simulink model "ISController"  (R2018a)
settings: Solver=FixedStepDiscrete  StartTime=0.0  StopTime=12  FixedStep=0.001  RelTol=1e-3  EnableMultiTasking=on
values from neighbouring files (symbols this model uses):
  Bx_ash_f = 11.7    [ISData.m]    (also in pacjeka_params.m)
  Bx_ash_r = 11.1    [ISData.m]    (also in pacjeka_params.m)
  Bx_snow_f = 10.2    [ISData.m]    (also in pacjeka_params.m)
  Bx_snow_r = 9.71    [ISData.m]    (also in pacjeka_params.m)
  By_ash_f = 8.86    [ISData.m]    (also in pacjeka_params.m)
  By_ash_r = 9.30    (= 9.3)    [ISData.m]    (also in pacjeka_params.m)
  By_snow_f = 19.1    [ISData.m]    (also in pacjeka_params.m)
  By_snow_r = 20.0    (= 20)    [ISData.m]    (also in pacjeka_params.m)
  Cx_ash_f = 1.69    [ISData.m]    (also in pacjeka_params.m)
  Cx_ash_r = 1.69    [ISData.m]    (also in pacjeka_params.m)
  Cx_snow_f = 1.96    [ISData.m]    (also in pacjeka_params.m)
  Cx_snow_r = 1.96    [ISData.m]    (also in pacjeka_params.m)
  Cy_ash_f = 1.19    [ISData.m]    (also in pacjeka_params.m)
  Cy_ash_r = 1.19    [ISData.m]    (also in pacjeka_params.m)
  Cy_snow_f = 0.550    (= 0.55)    [ISData.m]    (also in pacjeka_params.m)
  Cy_snow_r = 0.550    (= 0.55)    [ISData.m]    (also in pacjeka_params.m)
  D_phi = 16000    [ISData.m]    (also in IS_2impulse.m; IS_3impulse.m; IS_4impulse.m; InputShaper.m)
  D_theta = 30960    [ISData.m]    (also in IS_2impulse.m; IS_3impulse.m; IS_4impulse.m; InputShaper.m)
  delta_r = 0    [ISData.m]    (also in IS_2impulse.m; IS_3impulse.m; IS_4impulse.m; InputShaper.m)
  DLCTest = [0 0 0 0 0 0 0 0 0 0 0 0 ... (12003 elements, 12003x1)]    [DLCTest.mat]
  epsilon = 0.4    [ISData.m]    (also in IS_2impulse.m; IS_3impulse.m; IS_4impulse.m; InputShaper.m)
  Ex_ash_f = 0.377    [ISData.m]    (also in pacjeka_params.m)
  Ex_ash_r = 0.362    [ISData.m]    (also in pacjeka_params.m)
  Ex_snow_f = 0.651    [ISData.m]    (also in pacjeka_params.m)
  Ex_snow_r = 0.624    [ISData.m]    (also in pacjeka_params.m)
  Ey_ash_f = -1.21    [ISData.m]    (also in pacjeka_params.m)
  Ey_ash_r = -1.11    [ISData.m]    (also in pacjeka_params.m)
  Ey_snow_f = -2.1    [ISData.m]    (also in pacjeka_params.m)
  Ey_snow_r = -1.93    [ISData.m]    (also in pacjeka_params.m)
  g = 9.81    [ISData.m]    (also in IS_2impulse.m; IS_3impulse.m; IS_4impulse.m; InputShaper.m)
  h = 0.5    [ISData.m]    (also in IS_2impulse.m; IS_3impulse.m; IS_4impulse.m; InputShaper.m)
  Iw = 4    [ISData.m]    (also in IS_2impulse.m; IS_3impulse.m; IS_4impulse.m; InputShaper.m)
  Ixx = 602.1923    [ISData.m]    (also in IS_2impulse.m; IS_3impulse.m; IS_4impulse.m; InputShaper.m)
  Iyy = 2.7370e+03    (= 2737)    [ISData.m]    (also in IS_2impulse.m; IS_3impulse.m; IS_4impulse.m; InputShaper.m)
  Izz = 3070    [ISData.m]    (also in IS_2impulse.m; IS_3impulse.m; IS_4impulse.m; InputShaper.m)
  K_phi = 178000    [ISData.m]    (also in IS_2impulse.m; IS_3impulse.m; IS_4impulse.m; InputShaper.m)
  K_theta = 363540    [ISData.m]    (also in IS_2impulse.m; IS_3impulse.m; IS_4impulse.m; InputShaper.m)
  l_f = 1.2110    (= 1.211)    [ISData.m]    (also in IS_2impulse.m; IS_3impulse.m; IS_4impulse.m; InputShaper.m)
  l_r = 1.4590    (= 1.459)    [ISData.m]    (also in IS_2impulse.m; IS_3impulse.m; IS_4impulse.m; InputShaper.m)
  m = 1830    [ISData.m]    (also in IS_2impulse.m; IS_3impulse.m; IS_4impulse.m; InputShaper.m)
  mu_x_ash_f = 1.20    (= 1.2)    [ISData.m]    (also in pacjeka_params.m)
  mu_x_ash_r = 1.20    (= 1.2)    [ISData.m]    (also in pacjeka_params.m)
  mu_x_snow_f = 0.407    [ISData.m]    (also in pacjeka_params.m)
  mu_x_snow_r = 0.409    [ISData.m]    (also in pacjeka_params.m)
  mu_y_ash_f = 0.935    [ISData.m]    (also in pacjeka_params.m)
  mu_y_ash_r = 0.961    [ISData.m]    (also in pacjeka_params.m)
  mu_y_snow_f = 0.383    [ISData.m]    (also in pacjeka_params.m)
  mu_y_snow_r = 0.394    [ISData.m]    (also in pacjeka_params.m)
  omega0 = Vx0/Rw    (= 64.7813411079)    [ISData.m]    (also in IS_2impulse.m = 74.1; IS_3impulse.m = 74.1; IS_4impulse.m = 74.1; InputShaper.m = 74.0666666667)
  road = 1    [ISData.m]    (also in IS_2impulse.m; IS_3impulse.m; IS_4impulse.m; InputShaper.m)
  Rw = 0.3430    (= 0.343)    [ISData.m]    (also in IS_2impulse.m = 0.3; IS_3impulse.m = 0.3; IS_4impulse.m = 0.3; InputShaper.m = 0.3)
  thetaSW_actual = [thetaSW_actual, deltaSW]    [IS_2impulse.m]    (also in InputShaper.m; InputShaper2.m; thetaSW_IS_L.mat = [0 0 0 0 0 0 0 0 0 0 0 0 ... (12003 elements, 1x12003)]; thetaSW_IS_NL.mat = [0 0 0 0 0 0 0 0 0 0 0 0 ... (12003 elements, 1x12003)])
  Ts = 0.001    [ISData.m]    (also in IS_2impulse.m; IS_3impulse.m; IS_4impulse.m; InputShaper.m)
  Tsmall = 0.001    [ISData.m]    (also in IS_2impulse.m; IS_3impulse.m; IS_4impulse.m; InputShaper.m)
  Vx0 = 22.22    [ISData.m]    (also in IS_2impulse.m = states(3); IS_3impulse.m = states(3); IS_4impulse.m = states(3); InputShaper.m = states(3))
  w = 0.7700    (= 0.77)    [ISData.m]    (also in IS_2impulse.m; IS_3impulse.m; IS_4impulse.m; InputShaper.m)
libraries: simulink x2
(part 1 of 4)
settings Model: ExtModeTrigDuration=10000  Creator=srivats  LastModifiedBy=srivats
settings SolverCC: PositivePriorityOrder=on
settings RTWCC: SystemTargetFile=quarc_win64.tlc  TemplateMakefile=quarc_default_tmf  Description=QUARC Win64 Target
settings STFCustomTargetCC: TargetPreCompLibLocation=C:\PROGRA~3\QUARC\lib\2018a\win64\release  TargetLangStandard=C99 (ISO)  ConcurrentExecutionCompliant=on  SystemTargetFile=quarc_win64.tlc
settings GRTTargetCC: TargetPreCompLibLocation=C:\PROGRA~3\QUARC\lib\2018a\win64\release  ParMdlRefBuildCompliant=off  CompOptLevelCompliant=off  CombineOutputUpdateFcns=off  MatFileLogging=off  CPPClassGenCompliant=off  GRTInterface=on  UseToolchainInfoCompliant=off  ExtMode=on  ExtModeMexFile=quarc_comm

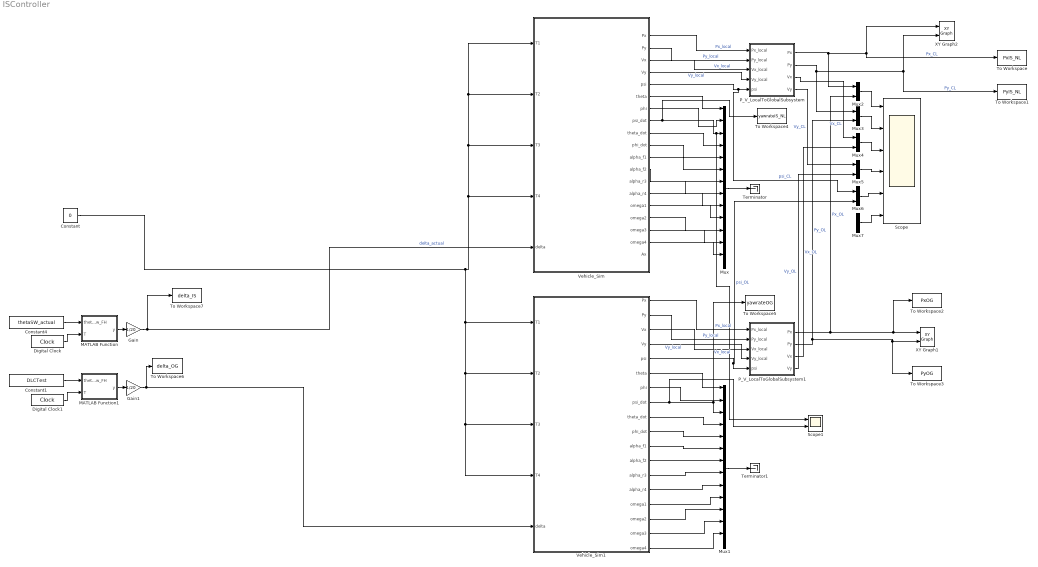
== system ISController ==
  Constant : Constant  Value=0
  Constant1 : Constant  Value=DLCTest
  Constant4 : Constant  Value=thetaSW_actual
  Digital Clock : DigitalClock  SampleTime=0.001
  Digital Clock1 : DigitalClock  SampleTime=0.001
  Gain : Gain  Gain=1/20
  Gain1 : Gain  Gain=1/20
  MATLAB Function : MATLAB Function  TreatAsAtomicUnit=on
  MATLAB Function1 : MATLAB Function  TreatAsAtomicUnit=on
  Mux : Mux  Inputs=14
  Mux1 : Mux  Inputs=14
  Mux{2..7} (6 alike) : Mux  Inputs=2
  P_V_LocalToGlobalSubsystem : Subsystem
  P_V_LocalToGlobalSubsystem1 : Subsystem
  Scope : Scope  NumInputPorts=6
  Scope1 : Scope  NumInputPorts=2
  Terminator : Terminator
  Terminator1 : Terminator
  To Workspace : ToWorkspace  VariableName=PxIS_NL  SaveFormat=Timeseries  SampleTime=-1
  To Workspace1 : ToWorkspace  VariableName=PyIS_NL  SaveFormat=Timeseries  SampleTime=-1
  To Workspace2 : ToWorkspace  VariableName=PxOG  SaveFormat=Timeseries  SampleTime=-1
  To Workspace3 : ToWorkspace  VariableName=PyOG  SaveFormat=Timeseries  SampleTime=-1
  To Workspace4 : ToWorkspace  VariableName=yawrateIS_NL  SaveFormat=Timeseries  SampleTime=-1
  To Workspace5 : ToWorkspace  VariableName=yawrateOG  SaveFormat=Timeseries  SampleTime=-1
  To Workspace6 : ToWorkspace  VariableName=delta_OG  SaveFormat=Timeseries  SampleTime=-1
  To Workspace7 : ToWorkspace  VariableName=delta_IS  SaveFormat=Timeseries  SampleTime=-1
  Vehicle_Sim : Subsystem
  Vehicle_Sim1 : Subsystem
  XY Graph1 : simulink/Sinks/XY Graph  xmin=0  xmax=700  ymin=-10  ymax=10  st=-1
  XY Graph2 : simulink/Sinks/XY Graph  xmin=0  xmax=700  ymin=-10  ymax=10  st=-1
  wires:
  Constant4/1 -> MATLAB Function/1(theta_sw_FH)
  Digital Clock/1 -> MATLAB Function/2(T)
  Vehicle_Sim1/10(phi_dot) -> Mux1/5
  Vehicle_Sim1/18(omega4) -> Mux1/13
  Vehicle_Sim1/7(phi) -> Mux1/2
  Vehicle_Sim/10(phi_dot) -> Mux/5
  Mux4/1 -> Scope/3
  Mux5/1 -> Scope/4
  P_V_LocalToGlobalSubsystem/4(Vy) -> Mux5/1  "Vy_CL"
  P_V_LocalToGlobalSubsystem1/3(Vx) -> Mux4/2  "Vx_OL"
  Mux2/1 -> Scope/1
  Vehicle_Sim1/15(omega1) -> Mux1/10
  Mux7/1 -> Scope/6
  Vehicle_Sim/17(omega3) -> Mux/12
  Mux6/1 -> Scope/5
  Vehicle_Sim1/14(alpha_r4) -> Mux1/9
  P_V_LocalToGlobalSubsystem1/2(Py) -> XY Graph1/2, To Workspace3/1, Mux3/2  "Py_OL"
  P_V_LocalToGlobalSubsystem1/4(Vy) -> Mux5/2  "Vy_OL"
  Vehicle_Sim/8(psi_dot) -> To Workspace4/1, Scope1/1, Mux/3
  Mux3/1 -> Scope/2
  P_V_LocalToGlobalSubsystem1/1(Px) -> Mux2/2, To Workspace2/1, XY Graph1/1  "Px_OL"
  Vehicle_Sim1/5(psi) -> Mux6/2, P_V_LocalToGlobalSubsystem1/5(psi)  "psi_OL"
  Vehicle_Sim1/12(alpha_f2) -> Mux1/7
  Vehicle_Sim/9(theta_dot) -> Mux/4
  Vehicle_Sim1/16(omega2) -> Mux1/11
  Vehicle_Sim/13(alpha_r3) -> Mux/8
  P_V_LocalToGlobalSubsystem/1(Px) -> XY Graph2/1, To Workspace/1, Mux2/1  "Px_CL"
  Constant/1 -> Vehicle_Sim1/4(T4), Vehicle_Sim1/3(T3), Vehicle_Sim1/2(T2), Vehicle_Sim1/1(T1), Vehicle_Sim/2(T2), Vehicle_Sim/1(T1), Vehicle_Sim/3(T3), Vehicle_Sim/4(T4)
  Vehicle_Sim/18(omega4) -> Mux/13
  Vehicle_Sim1/8(psi_dot) -> Scope1/2, To Workspace5/1, Mux1/3
  Mux1/1 -> Terminator1/1
  Vehicle_Sim/12(alpha_f2) -> Mux/7
  Vehicle_Sim1/17(omega3) -> Mux1/12
  Vehicle_Sim/16(omega2) -> Mux/11
  Vehicle_Sim1/6(theta) -> Mux1/1
  Vehicle_Sim1/13(alpha_r3) -> Mux1/8
  Vehicle_Sim1/4(Vy) -> P_V_LocalToGlobalSubsystem1/4(Vy_local)  "Vy_local"
  Vehicle_Sim1/2(Py) -> P_V_LocalToGlobalSubsystem1/2(Py_local)  "Py_local"
  Vehicle_Sim/3(Vx) -> P_V_LocalToGlobalSubsystem/3(Vx_local)  "Vx_local"
  Vehicle_Sim/5(psi) -> Mux6/1, P_V_LocalToGlobalSubsystem/5(psi)  "psi_CL"
  Vehicle_Sim/1(Px) -> P_V_LocalToGlobalSubsystem/1(Px_local)  "Px_local"
  Mux/1 -> Terminator/1
  P_V_LocalToGlobalSubsystem/2(Py) -> XY Graph2/2, To Workspace1/1, Mux3/1  "Py_CL"
  Vehicle_Sim/7(phi) -> Mux/2
  Vehicle_Sim1/3(Vx) -> P_V_LocalToGlobalSubsystem1/3(Vx_local)  "Vx_local"
  Vehicle_Sim/14(alpha_r4) -> Mux/9
  Vehicle_Sim1/11(alpha_f1) -> Mux1/6
  Vehicle_Sim/2(Py) -> P_V_LocalToGlobalSubsystem/2(Py_local)  "Py_local"
  P_V_LocalToGlobalSubsystem/3(Vx) -> Mux4/1  "Vx_CL"
  Vehicle_Sim/15(omega1) -> Mux/10
  Vehicle_Sim1/1(Px) -> P_V_LocalToGlobalSubsystem1/1(Px_local)  "Px_local"
  Vehicle_Sim1/9(theta_dot) -> Mux1/4
  Vehicle_Sim/4(Vy) -> P_V_LocalToGlobalSubsystem/4(Vy_local)  "Vy_local"
  Vehicle_Sim/6(theta) -> Mux/1
  Vehicle_Sim/11(alpha_f1) -> Mux/6
  MATLAB Function/1(y) -> Gain/1
  Gain/1 -> To Workspace7/1, Vehicle_Sim/5("delta ")  "delta_actual"
  MATLAB Function1/1(y) -> Gain1/1
  Constant1/1 -> MATLAB Function1/1(theta_sw_FH)
  Digital Clock1/1 -> MATLAB Function1/2(T)
  Gain1/1 -> To Workspace6/1, Vehicle_Sim1/5("delta ")

== system ISController/P_V_LocalToGlobalSubsystem ==
  Px_local : Inport  OutDataTypeStr=double  SampleTime=Ts
  Py_local : Inport  Port=2  OutDataTypeStr=double  SampleTime=Ts
  Vx_local : Inport  Port=3  OutDataTypeStr=double  SampleTime=Ts
  Vy_local : Inport  Port=4  OutDataTypeStr=double  SampleTime=Ts
  psi : Inport  Port=5  OutDataTypeStr=double  SampleTime=Ts
  Add : Sum  Inputs=+-
  Add1 : Sum
  Add2 : Sum  Inputs=+-
  Add3 : Sum
  Cos : Trigonometry  Operator=cos
  Product{,1..7} (8 alike) : Product
  Sin : Trigonometry
  Px : Outport  OutDataTypeStr=double  SampleTime=Ts
  Py : Outport  Port=2  OutDataTypeStr=double  SampleTime=Ts
  Vx : Outport  Port=3  OutDataTypeStr=double  SampleTime=Ts
  Vy : Outport  Port=4  OutDataTypeStr=double  SampleTime=Ts
  wires:
  Px_local/1 -> Product6/1, Product4/1  "Px_local"
  Py_local/1 -> Product7/1, Product5/1  "Py_local"
  Vx_local/1 -> Product2/1, Product/2  "Vx_local"
  Product5/1 -> Add2/2
  Product4/1 -> Add2/1
  Add2/1 -> Px/1  "Px"
  Product7/1 -> Add3/2
  Vy_local/1 -> Product3/1, Product1/2  "Vy_local"
  psi/1 -> Sin/1, Cos/1  "psi"
  Cos/1 -> Product3/2, Product/1, Product7/2, Product4/2  "cosPsi"
  Add3/1 -> Py/1  "Py"
  Product2/1 -> Add1/1
  Product1/1 -> Add/2
  Add/1 -> Vx/1  "Vx"
  Add1/1 -> Vy/1  "Vy"
  Product6/1 -> Add3/1
  Product3/1 -> Add1/2
  Product/1 -> Add/1
  Sin/1 -> Product2/2, Product1/1, Product6/2, Product5/2  "sinPsi"

== system ISController/P_V_LocalToGlobalSubsystem1 ==
  Px_local : Inport  OutDataTypeStr=double  SampleTime=Ts
  Py_local : Inport  Port=2  OutDataTypeStr=double  SampleTime=Ts
  Vx_local : Inport  Port=3  OutDataTypeStr=double  SampleTime=Ts
  Vy_local : Inport  Port=4  OutDataTypeStr=double  SampleTime=Ts
  psi : Inport  Port=5  OutDataTypeStr=double  SampleTime=Ts
  Add : Sum  Inputs=+-
  Add1 : Sum
  Add2 : Sum  Inputs=+-
  Add3 : Sum
  Cos : Trigonometry  Operator=cos
  Product{,1..7} (8 alike) : Product
  Sin : Trigonometry
  Px : Outport  OutDataTypeStr=double  SampleTime=Ts
  Py : Outport  Port=2  OutDataTypeStr=double  SampleTime=Ts
  Vx : Outport  Port=3  OutDataTypeStr=double  SampleTime=Ts
  Vy : Outport  Port=4  OutDataTypeStr=double  SampleTime=Ts
  wires:
  Px_local/1 -> Product6/1, Product4/1  "Px_local"
  Py_local/1 -> Product7/1, Product5/1  "Py_local"
  Vx_local/1 -> Product2/1, Product/2  "Vx_local"
  Product5/1 -> Add2/2
  Product4/1 -> Add2/1
  Add2/1 -> Px/1  "Px"
  Product7/1 -> Add3/2
  Vy_local/1 -> Product3/1, Product1/2  "Vy_local"
  psi/1 -> Sin/1, Cos/1  "psi"
  Cos/1 -> Product3/2, Product/1, Product7/2, Product4/2  "cosPsi"
  Add3/1 -> Py/1  "Py"
  Product2/1 -> Add1/1
  Product1/1 -> Add/2
  Add/1 -> Vx/1  "Vx"
  Add1/1 -> Vy/1  "Vy"
  Product6/1 -> Add3/1
  Product3/1 -> Add1/2
  Product/1 -> Add/1
  Sin/1 -> Product2/2, Product1/1, Product6/2, Product5/2  "sinPsi"

== system ISController/Vehicle_Sim ==
  T1 : Inport  OutDataTypeStr=double  SampleTime=Ts
  T2 : Inport  Port=2  OutDataTypeStr=double  SampleTime=Ts
  T3 : Inport  Port=3  OutDataTypeStr=double  SampleTime=Ts
  T4 : Inport  Port=4  OutDataTypeStr=double  SampleTime=Ts
  "delta " : Inport  Port=5
  Add1 : Sum
  Add2 : Sum
  Delay2 : Delay  DelayLength=1  SampleTime=Tsmall
  Delay3 : Delay  DelayLength=1  SampleTime=Tsmall
  Demux : Demux  Outputs=11
  Demux1 : Demux
  Gain1 : Gain  Gain=Tsmall
  Gain2 : Gain  Gain=Tsmall
  Mux : Mux  Inputs=11
      settings: DisplayOption=signals
  Mux1 : Mux
      settings: DisplayOption=signals
  Vehicle_model : Subsystem
  Vx_delay : Delay  DelayLength=1  InitialCondition=Vx0  SampleTime=Tsmall
  omega_delay : Delay  DelayLength=1  InitialCondition=omega0*ones(4,1)  SampleTime=Tsmall
  otherstates_delay : Delay  DelayLength=1  InitialCondition=zeros(11,1)  SampleTime=Tsmall
  Px : Outport  OutDataTypeStr=double  SampleTime=Tsmall
  Py : Outport  Port=2  OutDataTypeStr=double  SampleTime=Tsmall
  Vx : Outport  Port=3  OutDataTypeStr=double  SampleTime=Tsmall
  Vy : Outport  Port=4  OutDataTypeStr=double  SampleTime=Tsmall
  psi : Outport  Port=5  OutDataTypeStr=double  SampleTime=Tsmall
  theta : Outport  Port=6  OutDataTypeStr=double  SampleTime=Tsmall
  phi : Outport  Port=7  OutDataTypeStr=double  SampleTime=Tsmall
  psi_dot : Outport  Port=8  OutDataTypeStr=double  SampleTime=Tsmall
  theta_dot : Outport  Port=9  OutDataTypeStr=double  SampleTime=Tsmall
  phi_dot : Outport  Port=10  OutDataTypeStr=double  SampleTime=Tsmall
  alpha_f1 : Outport  Port=11  OutDataTypeStr=double  SampleTime=Tsmall
  alpha_f2 : Outport  Port=12  OutDataTypeStr=double  SampleTime=Tsmall
  alpha_r3 : Outport  Port=13  OutDataTypeStr=double  SampleTime=Tsmall
  alpha_r4 : Outport  Port=14  OutDataTypeStr=double  SampleTime=Tsmall
  omega1 : Outport  Port=15  OutDataTypeStr=double  SampleTime=Tsmall
  omega2 : Outport  Port=16  OutDataTypeStr=double  SampleTime=Tsmall
  omega3 : Outport  Port=17  OutDataTypeStr=double  SampleTime=Tsmall
  omega4 : Outport  Port=18  OutDataTypeStr=double  SampleTime=Tsmall
  Ax : Outport  Port=19
  wires:
  Vehicle_model/14(theta_next) -> Mux/9  "theta_next"
  Vehicle_model/12(psi_next) -> Mux/7  "psi_next"
  Vehicle_model/11(psi_dot_next) -> Mux/6  "psi_dot_next"
  Vehicle_model/15(phi_dot_next) -> Mux/10  "phi_dot_next"
  Mux/1 -> otherstates_delay/1
  Vehicle_model/3(alpha_f1_next) -> Mux/2  "alpha_f1_next"
  Vehicle_model/5(alpha_r3_next) -> Mux/4  "alpha_r3_next"
  Vehicle_model/9(omega3_next) -> Mux1/3  "omega3_next"
  Vehicle_model/8(omega2_next) -> Mux1/2  "omega2_next"
  Vehicle_model/13(theta_dot_next) -> Mux/8  "theta_dot_next"
  Vehicle_model/4(alpha_f2_next) -> Mux/3  "alpha_f2_next"
  Vehicle_model/6(alpha_r4_next) -> Mux/5  "alpha_r4_next"
  Vehicle_model/10(omega4_next) -> Mux1/4  "omega4_next"
  Vehicle_model/1(Vx_next) -> Vx_delay/1  "Vx_next"
  Demux/1 -> Gain2/1, Vy/1, Vehicle_model/6(Vy_curr)
  Vehicle_model/7(omega1_next) -> Mux1/1  "omega1_next"
  Demux1/3 -> omega3/1, Vehicle_model/13(omega3_curr)
  Demux/5 -> Vehicle_model/10(alpha_r4_curr), alpha_r4/1
  Demux/8 -> theta_dot/1, Vehicle_model/17(theta_dot_curr)
  Vehicle_model/16(phi_next) -> Mux/11  "phi_next"
  Vehicle_model/2(Vy_next) -> Mux/1  "Vy_next"
  T1/1 -> Vehicle_model/1(T1)
  Add2/1 -> Delay3/1
  Delay3/1 -> Py/1, Add2/2  "Py_curr"
  Add1/1 -> Delay2/1  "Px_next"
  Delay2/1 -> Px/1, Add1/2  "Px_curr"
  Gain1/1 -> Add1/1
  Gain2/1 -> Add2/1
  T3/1 -> Vehicle_model/3(T3)
  T4/1 -> Vehicle_model/4(T4)
  T2/1 -> Vehicle_model/2(T2)
  otherstates_delay/1 -> Demux/1
  Demux/4 -> Vehicle_model/9(alpha_r3_curr), alpha_r3/1
  Demux/11 -> phi/1, Vehicle_model/19(phi_curr)
  Demux/2 -> Vehicle_model/7(alpha_f1_curr), alpha_f1/1
  Demux/3 -> Vehicle_model/8(alpha_f2_curr), alpha_f2/1
  Demux1/4 -> omega4/1, Vehicle_model/14(omega4_curr)
  Demux/7 -> psi/1, Vehicle_model/16(psi_curr)
  Demux/9 -> theta/1, Vehicle_model/18(theta_curr)
  Demux/10 -> phi_dot/1, Vehicle_model/20(phi_dot_curr)
  Demux/6 -> psi_dot/1, Vehicle_model/15(psi_dot_curr)
  Demux1/2 -> omega2/1, Vehicle_model/12(omega2_curr)
  Vx_delay/1 -> Vx/1, Vehicle_model/5(Vx_curr), Gain1/1
  Demux1/1 -> omega1/1, Vehicle_model/11(omega1_curr)
  Mux1/1 -> omega_delay/1
  omega_delay/1 -> Demux1/1
  "delta "/1 -> Vehicle_model/21(delta)
  Vehicle_model/17(Ax) -> Ax/1

== system ISController/Vehicle_Sim1 ==
  T1 : Inport  OutDataTypeStr=double  SampleTime=Ts
  T2 : Inport  Port=2  OutDataTypeStr=double  SampleTime=Ts
  T3 : Inport  Port=3  OutDataTypeStr=double  SampleTime=Ts
  T4 : Inport  Port=4  OutDataTypeStr=double  SampleTime=Ts
  "delta " : Inport  Port=5
  Add1 : Sum
  Add2 : Sum
  Delay2 : Delay  DelayLength=1  SampleTime=Tsmall
  Delay3 : Delay  DelayLength=1  SampleTime=Tsmall
  Demux : Demux  Outputs=11
  Demux1 : Demux
  Gain1 : Gain  Gain=Tsmall
  Gain2 : Gain  Gain=Tsmall
  Mux : Mux  Inputs=11
      settings: DisplayOption=signals
  Mux1 : Mux
      settings: DisplayOption=signals
  Vehicle_model : Subsystem
  Vx_delay : Delay  DelayLength=1  InitialCondition=Vx0  SampleTime=Tsmall
  omega_delay : Delay  DelayLength=1  InitialCondition=omega0*ones(4,1)  SampleTime=Tsmall
  otherstates_delay : Delay  DelayLength=1  InitialCondition=zeros(11,1)  SampleTime=Tsmall
  Px : Outport  OutDataTypeStr=double  SampleTime=Tsmall
  Py : Outport  Port=2  OutDataTypeStr=double  SampleTime=Tsmall
  Vx : Outport  Port=3  OutDataTypeStr=double  SampleTime=Tsmall
  Vy : Outport  Port=4  OutDataTypeStr=double  SampleTime=Tsmall
  psi : Outport  Port=5  OutDataTypeStr=double  SampleTime=Tsmall
  theta : Outport  Port=6  OutDataTypeStr=double  SampleTime=Tsmall
  phi : Outport  Port=7  OutDataTypeStr=double  SampleTime=Tsmall
  psi_dot : Outport  Port=8  OutDataTypeStr=double  SampleTime=Tsmall
  theta_dot : Outport  Port=9  OutDataTypeStr=double  SampleTime=Tsmall
  phi_dot : Outport  Port=10  OutDataTypeStr=double  SampleTime=Tsmall
  alpha_f1 : Outport  Port=11  OutDataTypeStr=double  SampleTime=Tsmall
  alpha_f2 : Outport  Port=12  OutDataTypeStr=double  SampleTime=Tsmall
  alpha_r3 : Outport  Port=13  OutDataTypeStr=double  SampleTime=Tsmall
  alpha_r4 : Outport  Port=14  OutDataTypeStr=double  SampleTime=Tsmall
  omega1 : Outport  Port=15  OutDataTypeStr=double  SampleTime=Tsmall
  omega2 : Outport  Port=16  OutDataTypeStr=double  SampleTime=Tsmall
  omega3 : Outport  Port=17  OutDataTypeStr=double  SampleTime=Tsmall
  omega4 : Outport  Port=18  OutDataTypeStr=double  SampleTime=Tsmall
  wires:
  Vehicle_model/14(theta_next) -> Mux/9  "theta_next"
  Vehicle_model/12(psi_next) -> Mux/7  "psi_next"
  Vehicle_model/11(psi_dot_next) -> Mux/6  "psi_dot_next"
  Vehicle_model/15(phi_dot_next) -> Mux/10  "phi_dot_next"
  Mux/1 -> otherstates_delay/1
  Vehicle_model/3(alpha_f1_next) -> Mux/2  "alpha_f1_next"
  Vehicle_model/5(alpha_r3_next) -> Mux/4  "alpha_r3_next"
  Vehicle_model/9(omega3_next) -> Mux1/3  "omega3_next"
  Vehicle_model/8(omega2_next) -> Mux1/2  "omega2_next"
  Vehicle_model/13(theta_dot_next) -> Mux/8  "theta_dot_next"
  Vehicle_model/4(alpha_f2_next) -> Mux/3  "alpha_f2_next"
  Vehicle_model/6(alpha_r4_next) -> Mux/5  "alpha_r4_next"
  Vehicle_model/10(omega4_next) -> Mux1/4  "omega4_next"
  Vehicle_model/1(Vx_next) -> Vx_delay/1  "Vx_next"
  Demux/1 -> Gain2/1, Vy/1, Vehicle_model/6(Vy_curr)
  Vehicle_model/7(omega1_next) -> Mux1/1  "omega1_next"
  Demux1/3 -> omega3/1, Vehicle_model/13(omega3_curr)
  Demux/5 -> Vehicle_model/10(alpha_r4_curr), alpha_r4/1
  Demux/8 -> theta_dot/1, Vehicle_model/17(theta_dot_curr)
  Vehicle_model/16(phi_next) -> Mux/11  "phi_next"
  Vehicle_model/2(Vy_next) -> Mux/1  "Vy_next"
  T1/1 -> Vehicle_model/1(T1)
  Add2/1 -> Delay3/1
  Delay3/1 -> Py/1, Add2/2  "Py_curr"
  Add1/1 -> Delay2/1  "Px_next"
  Delay2/1 -> Px/1, Add1/2  "Px_curr"
  Gain1/1 -> Add1/1
  Gain2/1 -> Add2/1
  T3/1 -> Vehicle_model/3(T3)
  T4/1 -> Vehicle_model/4(T4)
  T2/1 -> Vehicle_model/2(T2)
  otherstates_delay/1 -> Demux/1
  Demux/4 -> Vehicle_model/9(alpha_r3_curr), alpha_r3/1
  Demux/11 -> phi/1, Vehicle_model/19(phi_curr)
  Demux/2 -> Vehicle_model/7(alpha_f1_curr), alpha_f1/1
  Demux/3 -> Vehicle_model/8(alpha_f2_curr), alpha_f2/1
  Demux1/4 -> omega4/1, Vehicle_model/14(omega4_curr)
  Demux/7 -> psi/1, Vehicle_model/16(psi_curr)
  Demux/9 -> theta/1, Vehicle_model/18(theta_curr)
  Demux/10 -> phi_dot/1, Vehicle_model/20(phi_dot_curr)
  Demux/6 -> psi_dot/1, Vehicle_model/15(psi_dot_curr)
  Demux1/2 -> omega2/1, Vehicle_model/12(omega2_curr)
  Vx_delay/1 -> Vx/1, Vehicle_model/5(Vx_curr), Gain1/1
  Demux1/1 -> omega1/1, Vehicle_model/11(omega1_curr)
  Mux1/1 -> omega_delay/1
  omega_delay/1 -> Demux1/1
  "delta "/1 -> Vehicle_model/21(delta)

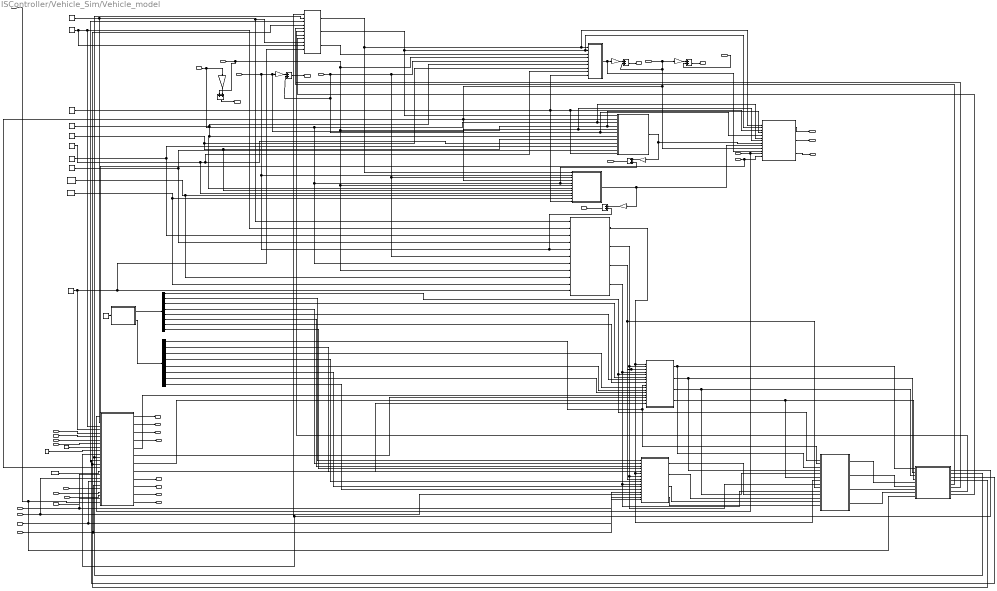
== system ISController/Vehicle_Sim/Vehicle_model ==
  T1 : Inport  OutDataTypeStr=double  SampleTime=Ts
  T2 : Inport  Port=2  OutDataTypeStr=double  SampleTime=Ts
  T3 : Inport  Port=3  OutDataTypeStr=double  SampleTime=Ts
  T4 : Inport  Port=4  OutDataTypeStr=double  SampleTime=Ts
  Vx_curr : Inport  Port=5  OutDataTypeStr=double  SampleTime=Tsmall
  Vy_curr : Inport  Port=6  OutDataTypeStr=double  SampleTime=Tsmall
  alpha_f1_curr : Inport  Port=7  OutDataTypeStr=double  SampleTime=Tsmall
  alpha_f2_curr : Inport  Port=8  OutDataTypeStr=double  SampleTime=Tsmall
  alpha_r3_curr : Inport  Port=9  OutDataTypeStr=double  SampleTime=Tsmall
  alpha_r4_curr : Inport  Port=10  OutDataTypeStr=double  SampleTime=Tsmall
  omega1_curr : Inport  Port=11  OutDataTypeStr=double  SampleTime=Tsmall
  omega2_curr : Inport  Port=12  OutDataTypeStr=double  SampleTime=Tsmall
  omega3_curr : Inport  Port=13  OutDataTypeStr=double  SampleTime=Tsmall
  omega4_curr : Inport  Port=14  OutDataTypeStr=double  SampleTime=Tsmall
  psi_dot_curr : Inport  Port=15  OutDataTypeStr=double  SampleTime=Tsmall
  psi_curr : Inport  Port=16  OutDataTypeStr=double  SampleTime=Tsmall
  theta_dot_curr : Inport  Port=17  OutDataTypeStr=double  SampleTime=Tsmall
  theta_curr : Inport  Port=18  OutDataTypeStr=double  SampleTime=Tsmall
  phi_curr : Inport  Port=19  OutDataTypeStr=double  SampleTime=Tsmall
  phi_dot_curr : Inport  Port=20  OutDataTypeStr=double  SampleTime=Tsmall
  delta : Inport  Port=21  OutDataTypeStr=double  SampleTime=Tsmall
  Add{,1..5} (6 alike) : Sum
  D_phi : Constant  Value=D_phi
  D_theta : Constant  Value=D_theta
  Demux1 : Demux  Outputs=8
  Demux2 : Demux  Outputs=8
  F_M_subsystem : Subsystem
  Fx0_Subsystem : Subsystem
  Fy0_Subsystem : Subsystem
  Fy0_to_Fy_subsystem : Subsystem
  Fz_Subsystem : Subsystem
  Gain{,1..5} (6 alike) : Gain  Gain=Tsmall
  Iw : Constant  Value=Iw
  Ixx : Constant  Value=Ixx
  Iyy : Constant  Value=Iyy
  Izz : Constant  Value=Izz
  K_phi : Constant  Value=K_phi
  K_theta : Constant  Value=K_theta
  Pacjeka_parameters_Subsystem : Subsystem
  Rw : Constant  Value=Rw
  Vx_Vy_Subsystem : Subsystem
  epsilon : Constant  Value=epsilon
  h : Constant  Value=h
  l_f : Constant  Value=l_f
  l_r : Constant  Value=l_r
  local_to_global_Fx_Fy_Subsystem : Subsystem
  omega_alpha_and_k_values_subsystem : Subsystem
  phi_subsystem : Subsystem
  psi_subsystem : Subsystem
  surface : Constant  Value=road
  theta_subsystem : Subsystem
  w : Constant  Value=w
  Vx_next : Outport  OutDataTypeStr=double  SampleTime=Tsmall
  Vy_next : Outport  Port=2  OutDataTypeStr=double  SampleTime=Tsmall
  alpha_f1_next : Outport  Port=3  OutDataTypeStr=double  SampleTime=Tsmall
  alpha_f2_next : Outport  Port=4  OutDataTypeStr=double  SampleTime=Tsmall
  alpha_r3_next : Outport  Port=5  OutDataTypeStr=double  SampleTime=Tsmall
  alpha_r4_next : Outport  Port=6  OutDataTypeStr=double  SampleTime=Tsmall
  omega1_next : Outport  Port=7  OutDataTypeStr=double  SampleTime=Tsmall
  omega2_next : Outport  Port=8  OutDataTypeStr=double  SampleTime=Tsmall
  omega3_next : Outport  Port=9  OutDataTypeStr=double  SampleTime=Tsmall
  omega4_next : Outport  Port=10  OutDataTypeStr=double  SampleTime=Tsmall
  psi_dot_next : Outport  Port=11  OutDataTypeStr=double  SampleTime=Tsmall
  psi_next : Outport  Port=12  OutDataTypeStr=double  SampleTime=Tsmall
  theta_dot_next : Outport  Port=13  OutDataTypeStr=double  SampleTime=Tsmall
  theta_next : Outport  Port=14  OutDataTypeStr=double  SampleTime=Tsmall
  phi_dot_next : Outport  Port=15  OutDataTypeStr=double  SampleTime=Tsmall
  phi_next : Outport  Port=16  OutDataTypeStr=double  SampleTime=Tsmall
  Ax : Outport  Port=17
  wires:
  Add/1 -> psi_dot_next/1
  Gain4/1 -> Add4/1
  Gain5/1 -> Add5/2
  Add4/1 -> phi_dot_next/1
  Add5/1 -> phi_next/1
  omega1_curr/1 -> omega_alpha_and_k_values_subsystem/22(omega1_curr)
  omega3_curr/1 -> omega_alpha_and_k_values_subsystem/24(omega3_curr)
  omega_alpha_and_k_values_subsystem/11(omega3_next) -> omega3_next/1
  omega_alpha_and_k_values_subsystem/12(omega4_next) -> omega4_next/1
  F_M_subsystem/2(FY) -> phi_subsystem/1(FY), Vx_Vy_Subsystem/2(FY), psi_subsystem/2(FY)  "Fy"
  theta_curr/1 -> Add3/2, Vx_Vy_Subsystem/5(theta), phi_subsystem/6(theta), psi_subsystem/5(theta), Fz_Subsystem/6(theta), theta_subsystem/3(theta)
  Ixx/1 -> psi_subsystem/6(Ixx), theta_subsystem/7(Ixx), phi_subsystem/7(Ixx)  "Ixx"
  phi_dot_curr/1 -> Vx_Vy_Subsystem/6(phi_dot), phi_subsystem/3(phi_dot), Add4/2, theta_subsystem/5(phi_dot), Fz_Subsystem/7(phi_dot), Gain5/1  "phi_dot"
  Izz/1 -> theta_subsystem/9(Izz), psi_subsystem/8(Izz), phi_subsystem/9(Izz)  "Izz"
  theta_subsystem/1(theta_ddot) -> Vx_Vy_Subsystem/9(theta_ddot), Gain2/1  "theta_ddot"
  K_phi/1 -> Fz_Subsystem/3(k_phi), phi_subsystem/10(K_phi)  "k_phi"
  F_M_subsystem/1(FX) -> theta_subsystem/1(FX), Vx_Vy_Subsystem/1(FX), psi_subsystem/1(FX)  "Fx"
  phi_curr/1 -> Add5/1, Fz_Subsystem/8(phi), theta_subsystem/6(phi), Vx_Vy_Subsystem/4(phi), phi_subsystem/4(phi), psi_subsystem/4(phi)
  theta_dot_curr/1 -> Gain3/1, Vx_Vy_Subsystem/7(theta_dot), phi_subsystem/5(theta_dot), theta_subsystem/2(theta_dot), Add2/2, Fz_Subsystem/5(theta_dot)
  F_M_subsystem/3(Mz) -> psi_subsystem/3(MZ)  "MZ"
  psi_subsystem/1(psi_ddot) -> Gain/1, Vx_Vy_Subsystem/11(psi_ddot)  "psi_ddot"
  phi_subsystem/1(phi_ddot) -> Vx_Vy_Subsystem/8(phi_ddot), Gain4/1  "phi_ddot"
  Iyy/1 -> psi_subsystem/7(Iyy), theta_subsystem/8(Iyy), phi_subsystem/8(Iyy)  "Iyy"
  D_theta/1 -> Fz_Subsystem/10(D_theta), theta_subsystem/11(D_theta)  "D_theta"
  Pacjeka_parameters_Subsystem/1(front) -> Demux1/1
  w/1 -> omega_alpha_and_k_values_subsystem/5(w), F_M_subsystem/11(w), Fz_Subsystem/11(w)  "w"
  Demux1/4 -> Fy0_Subsystem/2(C_y_f)  "C_y_f"
  Demux1/2 -> Fy0_Subsystem/1(mu_y_f)  "mu_y_f"
  Fz_Subsystem/2(Fz2) -> Fy0_to_Fy_subsystem/8(Fz2), Fy0_Subsystem/7(Fz2), Fx0_Subsystem/2(Fz2)  "Fz2"
  Demux2/1 -> Fy0_to_Fy_subsystem/2(mu_x_r), Fx0_Subsystem/9(mu_x_r)  "mu_x_r"
  omega_alpha_and_k_values_subsystem/6(k_f2) -> Fx0_Subsystem/14(k_f2)  "k_f2"
  Demux1/8 -> Fy0_Subsystem/4(E_y_f)  "E_y_f"
  Demux1/6 -> Fy0_Subsystem/3(B_y_f)  "B_y_f"
  surface/1 -> Pacjeka_parameters_Subsystem/1(surface_condition)
  l_r/1 -> F_M_subsystem/10(l_r), omega_alpha_and_k_values_subsystem/4(l_r), Fz_Subsystem/2(l_r)  "l_r"
  Fz_Subsystem/4(Fz4) -> Fy0_to_Fy_subsystem/10(Fz4), Fy0_Subsystem/10(Fz4), Fx0_Subsystem/4(Fz4)  "Fz4"
  Demux1/5 -> Fx0_Subsystem/7(B_x_f)  "B_x_f"
  Demux1/7 -> Fx0_Subsystem/8(E_x_f)  "E_x_f"
  D_phi/1 -> Fz_Subsystem/4(d_phi), phi_subsystem/11(D_phi)  "d_phi"
  omega_alpha_and_k_values_subsystem/5(k_f1) -> Fx0_Subsystem/13(k_f1)  "k_f1"
  Demux1/1 -> Fy0_to_Fy_subsystem/1(mu_x_f), Fx0_Subsystem/5(mu_x_f)  "mu_x_f"
  omega_alpha_and_k_values_subsystem/7(k_r3) -> Fx0_Subsystem/15(k_r3)  "k_r3"
  l_f/1 -> omega_alpha_and_k_values_subsystem/3(l_f), F_M_subsystem/9(l_f), Fz_Subsystem/1(l_f)  "l_f"
  K_theta/1 -> Fz_Subsystem/9(K_theta), theta_subsystem/10(K_theta)  "K_theta"
  Demux2/3 -> Fx0_Subsystem/10(C_x_r)  "C_x_r"
  Demux2/7 -> Fx0_Subsystem/12(E_x_r)  "E_x_r"
  Pacjeka_parameters_Subsystem/2(rear) -> Demux2/1
  omega_alpha_and_k_values_subsystem/8(k_r4) -> Fx0_Subsystem/16(k_r4)  "k_r4"
  Fx0_Subsystem/1(Fx01) -> local_to_global_Fx_Fy_Subsystem/1(local_Fx1), Fy0_to_Fy_subsystem/3(Fx01)  "Fx01"
  Demux1/3 -> Fx0_Subsystem/6(C_x_f)  "C_x_f"
  Demux2/5 -> Fx0_Subsystem/11(B_x_r)  "B_x_r"
  Fz_Subsystem/1(Fz1) -> Fx0_Subsystem/1(Fz1), Fy0_to_Fy_subsystem/7(Fz1), Fy0_Subsystem/6(Fz1)  "Fz1"
  Demux2/6 -> Fy0_Subsystem/11(B_y_r)  "B_y_r"
  Fz_Subsystem/3(Fz3) -> Fy0_to_Fy_subsystem/9(Fz3), Fx0_Subsystem/3(Fz3), Fy0_Subsystem/8(Fz3)  "Fz3"
  local_to_global_Fx_Fy_Subsystem/6(Fy2) -> F_M_subsystem/6(Fy2)  "Fy2"
  T4/1 -> omega_alpha_and_k_values_subsystem/9(T4)
  Demux2/8 -> Fy0_Subsystem/12(E_y_r)  "E_y_r"
  Fy0_Subsystem/4(Fy04) -> Fy0_to_Fy_subsystem/14(Fy04)  "Fy04"
  alpha_f1_curr/1 -> omega_alpha_and_k_values_subsystem/18(alpha_f1_curr), Fy0_Subsystem/13(alpha_f1)
  epsilon/1 -> omega_alpha_and_k_values_subsystem/17(epsilon)
  Vx_Vy_Subsystem/1(Vx_next) -> Vx_next/1
  Fx0_Subsystem/4(Fx04) -> local_to_global_Fx_Fy_Subsystem/4(local_Fx4), Fy0_to_Fy_subsystem/6(Fx04)  "Fx04"
  alpha_f2_curr/1 -> Fy0_Subsystem/14(alpha_f2), omega_alpha_and_k_values_subsystem/19(alpha_f2_curr)
  Fy0_Subsystem/1(Fy01) -> Fy0_to_Fy_subsystem/11(Fy01)  "Fy01"
  Fy0_Subsystem/2(Fy02) -> Fy0_to_Fy_subsystem/12(Fy02)  "Fy02"
  Demux2/4 -> Fy0_Subsystem/9(C_y_r)  "C_y_r"
  local_to_global_Fx_Fy_Subsystem/5(Fy1) -> F_M_subsystem/5(Fy1)  "Fy1"
  Fx0_Subsystem/3(Fx03) -> Fy0_to_Fy_subsystem/5(Fx03), local_to_global_Fx_Fy_Subsystem/3(local_Fx3)  "Fx03"
  local_to_global_Fx_Fy_Subsystem/7(Fy3) -> F_M_subsystem/7(Fy3)  "Fy3"
  Rw/1 -> omega_alpha_and_k_values_subsystem/10(Rw)
  h/1 -> Vx_Vy_Subsystem/3(h), phi_subsystem/12(h), psi_subsystem/9(h), theta_subsystem/12(h)  "h"
  Fx0_Subsystem/2(Fx02) -> local_to_global_Fx_Fy_Subsystem/2(local_Fx2), Fy0_to_Fy_subsystem/4(Fx02)
  local_to_global_Fx_Fy_Subsystem/8(Fy4) -> F_M_subsystem/8(Fy4)  "Fy4"
  T3/1 -> omega_alpha_and_k_values_subsystem/8(T3)
  T1/1 -> omega_alpha_and_k_values_subsystem/6(T1)
  Iw/1 -> omega_alpha_and_k_values_subsystem/11(Iw)
  T2/1 -> omega_alpha_and_k_values_subsystem/7(T2)
  alpha_r4_curr/1 -> Fy0_Subsystem/16(alpha_r4), omega_alpha_and_k_values_subsystem/21(alpha_r4_curr)
  Fy0_Subsystem/3(Fy03) -> Fy0_to_Fy_subsystem/13(Fy03)  "Fy03"
  Demux2/2 -> Fy0_Subsystem/5(mu_y_r)  "mu_y_r"
  alpha_r3_curr/1 -> Fy0_Subsystem/15(alpha_r3), omega_alpha_and_k_values_subsystem/20(alpha_r3_curr)
  Vy_curr/1 -> omega_alpha_and_k_values_subsystem/2(Vy), Vx_Vy_Subsystem/13(Vy_curr)
  omega_alpha_and_k_values_subsystem/3(alpha_r3_next) -> alpha_r3_next/1
  Vx_curr/1 -> omega_alpha_and_k_values_subsystem/1(Vx), Vx_Vy_Subsystem/12(Vx_curr)
  omega_alpha_and_k_values_subsystem/1(alpha_f1_next) -> alpha_f1_next/1  "alpha_f1"
  omega_alpha_and_k_values_subsystem/4(alpha_r4_next) -> alpha_r4_next/1  "alpha_r4"
  Vx_Vy_Subsystem/2(Vy_next) -> Vy_next/1
  omega_alpha_and_k_values_subsystem/2(alpha_f2_next) -> alpha_f2_next/1  "alpha_f2"
  psi_dot_curr/1 -> Gain1/1, Add/2, Vx_Vy_Subsystem/10(psi_dot), omega_alpha_and_k_values_subsystem/16(psi_dot), theta_subsystem/4(psi_dot), phi_subsystem/2(psi_dot)  "psi_dot"
  Gain1/1 -> Add1/1
  psi_curr/1 -> Add1/2
  omega4_curr/1 -> omega_alpha_and_k_values_subsystem/25(omega4_curr)
  omega_alpha_and_k_values_subsystem/10(omega2_next) -> omega2_next/1
  omega2_curr/1 -> omega_alpha_and_k_values_subsystem/23(omega2_curr)
  Gain3/1 -> Add3/1
  Gain2/1 -> Add2/1
  Gain/1 -> Add/1
  Add3/1 -> theta_next/1
  Add2/1 -> theta_dot_next/1
  Add1/1 -> psi_next/1
  omega_alpha_and_k_values_subsystem/9(omega1_next) -> omega1_next/1
  delta/1 -> local_to_global_Fx_Fy_Subsystem/9(delta_f2), omega_alpha_and_k_values_subsystem/26(delta_f2)  "delta_f2"
  Fy0_to_Fy_subsystem/1(local_Fy1) -> local_to_global_Fx_Fy_Subsystem/5(local_Fy1)  "Fy1"
  Fy0_to_Fy_subsystem/2(local_Fy2) -> local_to_global_Fx_Fy_Subsystem/6(local_Fy2)  "Fy2"
  Fy0_to_Fy_subsystem/3(local_Fy3) -> local_to_global_Fx_Fy_Subsystem/7(local_Fy3)  "Fy3"
  Fy0_to_Fy_subsystem/4(lcoal_Fy4) -> local_to_global_Fx_Fy_Subsystem/8(local_Fy4)  "Fy4"
  local_to_global_Fx_Fy_Subsystem/1(Fx1) -> omega_alpha_and_k_values_subsystem/12(Fx1), F_M_subsystem/1(Fx1)  "Fx1"
  local_to_global_Fx_Fy_Subsystem/2(Fx2) -> omega_alpha_and_k_values_subsystem/13(Fx2), F_M_subsystem/2(Fx2)  "Fx2"
  local_to_global_Fx_Fy_Subsystem/3(Fx3) -> F_M_subsystem/3(Fx3), omega_alpha_and_k_values_subsystem/14(Fx3)  "Fx3"
  local_to_global_Fx_Fy_Subsystem/4(Fx4) -> F_M_subsystem/4(Fx4), omega_alpha_and_k_values_subsystem/15(Fx4)  "Fx4"
  Vx_Vy_Subsystem/3(Ax) -> Ax/1

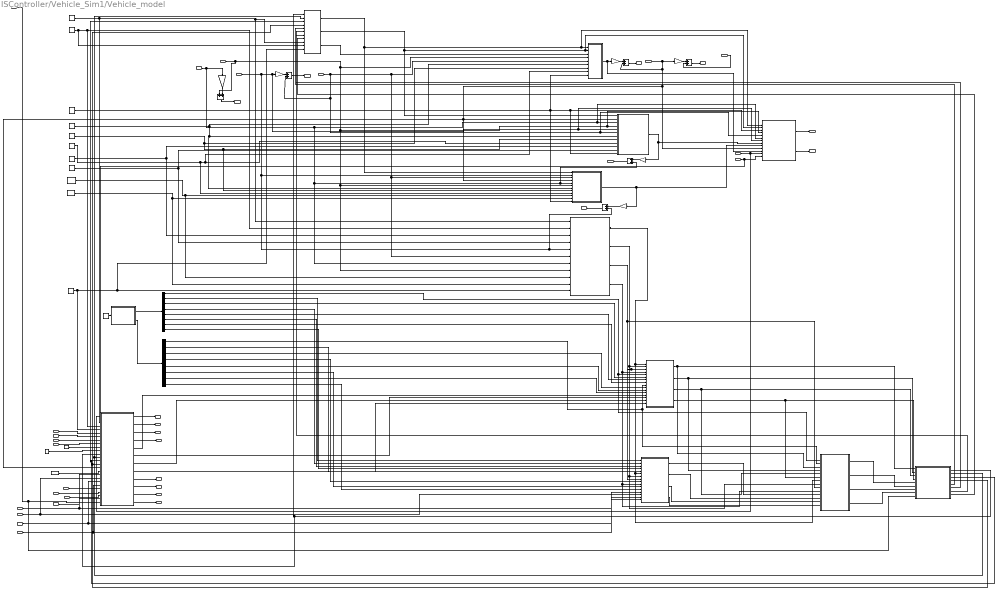
== system ISController/Vehicle_Sim1/Vehicle_model ==
  T1 : Inport  OutDataTypeStr=double  SampleTime=Ts
  T2 : Inport  Port=2  OutDataTypeStr=double  SampleTime=Ts
  T3 : Inport  Port=3  OutDataTypeStr=double  SampleTime=Ts
  T4 : Inport  Port=4  OutDataTypeStr=double  SampleTime=Ts
  Vx_curr : Inport  Port=5  OutDataTypeStr=double  SampleTime=Tsmall
  Vy_curr : Inport  Port=6  OutDataTypeStr=double  SampleTime=Tsmall
  alpha_f1_curr : Inport  Port=7  OutDataTypeStr=double  SampleTime=Tsmall
  alpha_f2_curr : Inport  Port=8  OutDataTypeStr=double  SampleTime=Tsmall
  alpha_r3_curr : Inport  Port=9  OutDataTypeStr=double  SampleTime=Tsmall
  alpha_r4_curr : Inport  Port=10  OutDataTypeStr=double  SampleTime=Tsmall
  omega1_curr : Inport  Port=11  OutDataTypeStr=double  SampleTime=Tsmall
  omega2_curr : Inport  Port=12  OutDataTypeStr=double  SampleTime=Tsmall
  omega3_curr : Inport  Port=13  OutDataTypeStr=double  SampleTime=Tsmall
  omega4_curr : Inport  Port=14  OutDataTypeStr=double  SampleTime=Tsmall
  psi_dot_curr : Inport  Port=15  OutDataTypeStr=double  SampleTime=Tsmall
  psi_curr : Inport  Port=16  OutDataTypeStr=double  SampleTime=Tsmall
  theta_dot_curr : Inport  Port=17  OutDataTypeStr=double  SampleTime=Tsmall
  theta_curr : Inport  Port=18  OutDataTypeStr=double  SampleTime=Tsmall
  phi_curr : Inport  Port=19  OutDataTypeStr=double  SampleTime=Tsmall
  phi_dot_curr : Inport  Port=20  OutDataTypeStr=double  SampleTime=Tsmall
  delta : Inport  Port=21  OutDataTypeStr=double  SampleTime=Tsmall
  Add{,1..5} (6 alike) : Sum
  D_phi : Constant  Value=D_phi
  D_theta : Constant  Value=D_theta
  Demux1 : Demux  Outputs=8
  Demux2 : Demux  Outputs=8
  F_M_subsystem : Subsystem
  Fx0_Subsystem : Subsystem
  Fy0_Subsystem : Subsystem
  Fy0_to_Fy_subsystem : Subsystem
  Fz_Subsystem : Subsystem
  Gain{,1..5} (6 alike) : Gain  Gain=Tsmall
  Iw : Constant  Value=Iw
  Ixx : Constant  Value=Ixx
  Iyy : Constant  Value=Iyy
  Izz : Constant  Value=Izz
  K_phi : Constant  Value=K_phi
  K_theta : Constant  Value=K_theta
  Pacjeka_parameters_Subsystem : Subsystem
  Rw : Constant  Value=Rw
  Vx_Vy_Subsystem : Subsystem
  epsilon : Constant  Value=epsilon
  h : Constant  Value=h
  l_f : Constant  Value=l_f
  l_r : Constant  Value=l_r
  local_to_global_Fx_Fy_Subsystem : Subsystem
  omega_alpha_and_k_values_subsystem : Subsystem
  phi_subsystem : Subsystem
  psi_subsystem : Subsystem
  surface : Constant  Value=road
  theta_subsystem : Subsystem
  w : Constant  Value=w
  Vx_next : Outport  OutDataTypeStr=double  SampleTime=Tsmall
  Vy_next : Outport  Port=2  OutDataTypeStr=double  SampleTime=Tsmall
  alpha_f1_next : Outport  Port=3  OutDataTypeStr=double  SampleTime=Tsmall
  alpha_f2_next : Outport  Port=4  OutDataTypeStr=double  SampleTime=Tsmall
  alpha_r3_next : Outport  Port=5  OutDataTypeStr=double  SampleTime=Tsmall
  alpha_r4_next : Outport  Port=6  OutDataTypeStr=double  SampleTime=Tsmall
  omega1_next : Outport  Port=7  OutDataTypeStr=double  SampleTime=Tsmall
  omega2_next : Outport  Port=8  OutDataTypeStr=double  SampleTime=Tsmall
  omega3_next : Outport  Port=9  OutDataTypeStr=double  SampleTime=Tsmall
  omega4_next : Outport  Port=10  OutDataTypeStr=double  SampleTime=Tsmall
  psi_dot_next : Outport  Port=11  OutDataTypeStr=double  SampleTime=Tsmall
  psi_next : Outport  Port=12  OutDataTypeStr=double  SampleTime=Tsmall
  theta_dot_next : Outport  Port=13  OutDataTypeStr=double  SampleTime=Tsmall
  theta_next : Outport  Port=14  OutDataTypeStr=double  SampleTime=Tsmall
  phi_dot_next : Outport  Port=15  OutDataTypeStr=double  SampleTime=Tsmall
  phi_next : Outport  Port=16  OutDataTypeStr=double  SampleTime=Tsmall
  wires:
  Add/1 -> psi_dot_next/1
  Gain4/1 -> Add4/1
  Gain5/1 -> Add5/2
  Add4/1 -> phi_dot_next/1
  Add5/1 -> phi_next/1
  omega1_curr/1 -> omega_alpha_and_k_values_subsystem/22(omega1_curr)
  omega3_curr/1 -> omega_alpha_and_k_values_subsystem/24(omega3_curr)
  omega_alpha_and_k_values_subsystem/11(omega3_next) -> omega3_next/1
  omega_alpha_and_k_values_subsystem/12(omega4_next) -> omega4_next/1
  F_M_subsystem/2(FY) -> phi_subsystem/1(FY), Vx_Vy_Subsystem/2(FY), psi_subsystem/2(FY)  "Fy"
  theta_curr/1 -> Add3/2, Vx_Vy_Subsystem/5(theta), phi_subsystem/6(theta), psi_subsystem/5(theta), Fz_Subsystem/6(theta), theta_subsystem/3(theta)
  Ixx/1 -> psi_subsystem/6(Ixx), theta_subsystem/7(Ixx), phi_subsystem/7(Ixx)  "Ixx"
  phi_dot_curr/1 -> Vx_Vy_Subsystem/6(phi_dot), phi_subsystem/3(phi_dot), Add4/2, theta_subsystem/5(phi_dot), Fz_Subsystem/7(phi_dot), Gain5/1  "phi_dot"
  Izz/1 -> theta_subsystem/9(Izz), psi_subsystem/8(Izz), phi_subsystem/9(Izz)  "Izz"
  theta_subsystem/1(theta_ddot) -> Vx_Vy_Subsystem/9(theta_ddot), Gain2/1  "theta_ddot"
  K_phi/1 -> Fz_Subsystem/3(k_phi), phi_subsystem/10(K_phi)  "k_phi"
  F_M_subsystem/1(FX) -> theta_subsystem/1(FX), Vx_Vy_Subsystem/1(FX), psi_subsystem/1(FX)  "Fx"
  phi_curr/1 -> Add5/1, Fz_Subsystem/8(phi), theta_subsystem/6(phi), Vx_Vy_Subsystem/4(phi), phi_subsystem/4(phi), psi_subsystem/4(phi)
  theta_dot_curr/1 -> Gain3/1, Vx_Vy_Subsystem/7(theta_dot), phi_subsystem/5(theta_dot), theta_subsystem/2(theta_dot), Add2/2, Fz_Subsystem/5(theta_dot)
  F_M_subsystem/3(Mz) -> psi_subsystem/3(MZ)  "MZ"
  psi_subsystem/1(psi_ddot) -> Gain/1, Vx_Vy_Subsystem/11(psi_ddot)  "psi_ddot"
  phi_subsystem/1(phi_ddot) -> Vx_Vy_Subsystem/8(phi_ddot), Gain4/1  "phi_ddot"
  Iyy/1 -> psi_subsystem/7(Iyy), theta_subsystem/8(Iyy), phi_subsystem/8(Iyy)  "Iyy"
  D_theta/1 -> Fz_Subsystem/10(D_theta), theta_subsystem/11(D_theta)  "D_theta"
  Pacjeka_parameters_Subsystem/1(front) -> Demux1/1
  w/1 -> omega_alpha_and_k_values_subsystem/5(w), F_M_subsystem/11(w), Fz_Subsystem/11(w)  "w"
  Demux1/4 -> Fy0_Subsystem/2(C_y_f)  "C_y_f"
  Demux1/2 -> Fy0_Subsystem/1(mu_y_f)  "mu_y_f"
  Fz_Subsystem/2(Fz2) -> Fy0_to_Fy_subsystem/8(Fz2), Fy0_Subsystem/7(Fz2), Fx0_Subsystem/2(Fz2)  "Fz2"
  Demux2/1 -> Fy0_to_Fy_subsystem/2(mu_x_r), Fx0_Subsystem/9(mu_x_r)  "mu_x_r"
  omega_alpha_and_k_values_subsystem/6(k_f2) -> Fx0_Subsystem/14(k_f2)  "k_f2"
  Demux1/8 -> Fy0_Subsystem/4(E_y_f)  "E_y_f"
  Demux1/6 -> Fy0_Subsystem/3(B_y_f)  "B_y_f"
  surface/1 -> Pacjeka_parameters_Subsystem/1(surface_condition)
  l_r/1 -> F_M_subsystem/10(l_r), omega_alpha_and_k_values_subsystem/4(l_r), Fz_Subsystem/2(l_r)  "l_r"
  Fz_Subsystem/4(Fz4) -> Fy0_to_Fy_subsystem/10(Fz4), Fy0_Subsystem/10(Fz4), Fx0_Subsystem/4(Fz4)  "Fz4"
  Demux1/5 -> Fx0_Subsystem/7(B_x_f)  "B_x_f"
  Demux1/7 -> Fx0_Subsystem/8(E_x_f)  "E_x_f"
  D_phi/1 -> Fz_Subsystem/4(d_phi), phi_subsystem/11(D_phi)  "d_phi"
  omega_alpha_and_k_values_subsystem/5(k_f1) -> Fx0_Subsystem/13(k_f1)  "k_f1"
  Demux1/1 -> Fy0_to_Fy_subsystem/1(mu_x_f), Fx0_Subsystem/5(mu_x_f)  "mu_x_f"
  omega_alpha_and_k_values_subsystem/7(k_r3) -> Fx0_Subsystem/15(k_r3)  "k_r3"
  l_f/1 -> omega_alpha_and_k_values_subsystem/3(l_f), F_M_subsystem/9(l_f), Fz_Subsystem/1(l_f)  "l_f"
  K_theta/1 -> Fz_Subsystem/9(K_theta), theta_subsystem/10(K_theta)  "K_theta"
  Demux2/3 -> Fx0_Subsystem/10(C_x_r)  "C_x_r"
  Demux2/7 -> Fx0_Subsystem/12(E_x_r)  "E_x_r"
  Pacjeka_parameters_Subsystem/2(rear) -> Demux2/1
  omega_alpha_and_k_values_subsystem/8(k_r4) -> Fx0_Subsystem/16(k_r4)  "k_r4"
  Fx0_Subsystem/1(Fx01) -> local_to_global_Fx_Fy_Subsystem/1(local_Fx1), Fy0_to_Fy_subsystem/3(Fx01)  "Fx01"
  Demux1/3 -> Fx0_Subsystem/6(C_x_f)  "C_x_f"
  Demux2/5 -> Fx0_Subsystem/11(B_x_r)  "B_x_r"
  Fz_Subsystem/1(Fz1) -> Fx0_Subsystem/1(Fz1), Fy0_to_Fy_subsystem/7(Fz1), Fy0_Subsystem/6(Fz1)  "Fz1"
  Demux2/6 -> Fy0_Subsystem/11(B_y_r)  "B_y_r"
  Fz_Subsystem/3(Fz3) -> Fy0_to_Fy_subsystem/9(Fz3), Fx0_Subsystem/3(Fz3), Fy0_Subsystem/8(Fz3)  "Fz3"
  local_to_global_Fx_Fy_Subsystem/6(Fy2) -> F_M_subsystem/6(Fy2)  "Fy2"
  T4/1 -> omega_alpha_and_k_values_subsystem/9(T4)
  Demux2/8 -> Fy0_Subsystem/12(E_y_r)  "E_y_r"
  Fy0_Subsystem/4(Fy04) -> Fy0_to_Fy_subsystem/14(Fy04)  "Fy04"
  alpha_f1_curr/1 -> omega_alpha_and_k_values_subsystem/18(alpha_f1_curr), Fy0_Subsystem/13(alpha_f1)
  epsilon/1 -> omega_alpha_and_k_values_subsystem/17(epsilon)
  Vx_Vy_Subsystem/1(Vx_next) -> Vx_next/1
  Fx0_Subsystem/4(Fx04) -> local_to_global_Fx_Fy_Subsystem/4(local_Fx4), Fy0_to_Fy_subsystem/6(Fx04)  "Fx04"
  alpha_f2_curr/1 -> Fy0_Subsystem/14(alpha_f2), omega_alpha_and_k_values_subsystem/19(alpha_f2_curr)
  Fy0_Subsystem/1(Fy01) -> Fy0_to_Fy_subsystem/11(Fy01)  "Fy01"
  Fy0_Subsystem/2(Fy02) -> Fy0_to_Fy_subsystem/12(Fy02)  "Fy02"
  Demux2/4 -> Fy0_Subsystem/9(C_y_r)  "C_y_r"
  local_to_global_Fx_Fy_Subsystem/5(Fy1) -> F_M_subsystem/5(Fy1)  "Fy1"
  Fx0_Subsystem/3(Fx03) -> Fy0_to_Fy_subsystem/5(Fx03), local_to_global_Fx_Fy_Subsystem/3(local_Fx3)  "Fx03"
  local_to_global_Fx_Fy_Subsystem/7(Fy3) -> F_M_subsystem/7(Fy3)  "Fy3"
  Rw/1 -> omega_alpha_and_k_values_subsystem/10(Rw)
  h/1 -> Vx_Vy_Subsystem/3(h), phi_subsystem/12(h), psi_subsystem/9(h), theta_subsystem/12(h)  "h"
  Fx0_Subsystem/2(Fx02) -> local_to_global_Fx_Fy_Subsystem/2(local_Fx2), Fy0_to_Fy_subsystem/4(Fx02)
  local_to_global_Fx_Fy_Subsystem/8(Fy4) -> F_M_subsystem/8(Fy4)  "Fy4"
  T3/1 -> omega_alpha_and_k_values_subsystem/8(T3)
  T1/1 -> omega_alpha_and_k_values_subsystem/6(T1)
  Iw/1 -> omega_alpha_and_k_values_subsystem/11(Iw)
  T2/1 -> omega_alpha_and_k_values_subsystem/7(T2)
  alpha_r4_curr/1 -> Fy0_Subsystem/16(alpha_r4), omega_alpha_and_k_values_subsystem/21(alpha_r4_curr)
  Fy0_Subsystem/3(Fy03) -> Fy0_to_Fy_subsystem/13(Fy03)  "Fy03"
  Demux2/2 -> Fy0_Subsystem/5(mu_y_r)  "mu_y_r"
  alpha_r3_curr/1 -> Fy0_Subsystem/15(alpha_r3), omega_alpha_and_k_values_subsystem/20(alpha_r3_curr)
  Vy_curr/1 -> omega_alpha_and_k_values_subsystem/2(Vy), Vx_Vy_Subsystem/13(Vy_curr)
  omega_alpha_and_k_values_subsystem/3(alpha_r3_next) -> alpha_r3_next/1
  Vx_curr/1 -> omega_alpha_and_k_values_subsystem/1(Vx), Vx_Vy_Subsystem/12(Vx_curr)
  omega_alpha_and_k_values_subsystem/1(alpha_f1_next) -> alpha_f1_next/1  "alpha_f1"
  omega_alpha_and_k_values_subsystem/4(alpha_r4_next) -> alpha_r4_next/1  "alpha_r4"
  Vx_Vy_Subsystem/2(Vy_next) -> Vy_next/1
  omega_alpha_and_k_values_subsystem/2(alpha_f2_next) -> alpha_f2_next/1  "alpha_f2"
  psi_dot_curr/1 -> Gain1/1, Add/2, Vx_Vy_Subsystem/10(psi_dot), omega_alpha_and_k_values_subsystem/16(psi_dot), theta_subsystem/4(psi_dot), phi_subsystem/2(psi_dot)  "psi_dot"
  Gain1/1 -> Add1/1
  psi_curr/1 -> Add1/2
  omega4_curr/1 -> omega_alpha_and_k_values_subsystem/25(omega4_curr)
  omega_alpha_and_k_values_subsystem/10(omega2_next) -> omega2_next/1
  omega2_curr/1 -> omega_alpha_and_k_values_subsystem/23(omega2_curr)
  Gain3/1 -> Add3/1
  Gain2/1 -> Add2/1
  Gain/1 -> Add/1
  Add3/1 -> theta_next/1
  Add2/1 -> theta_dot_next/1
  Add1/1 -> psi_next/1
  omega_alpha_and_k_values_subsystem/9(omega1_next) -> omega1_next/1
  delta/1 -> local_to_global_Fx_Fy_Subsystem/9(delta_f2), omega_alpha_and_k_values_subsystem/26(delta_f2)  "delta_f2"
  Fy0_to_Fy_subsystem/1(local_Fy1) -> local_to_global_Fx_Fy_Subsystem/5(local_Fy1)  "Fy1"
  Fy0_to_Fy_subsystem/2(local_Fy2) -> local_to_global_Fx_Fy_Subsystem/6(local_Fy2)  "Fy2"
  Fy0_to_Fy_subsystem/3(local_Fy3) -> local_to_global_Fx_Fy_Subsystem/7(local_Fy3)  "Fy3"
  Fy0_to_Fy_subsystem/4(lcoal_Fy4) -> local_to_global_Fx_Fy_Subsystem/8(local_Fy4)  "Fy4"
  local_to_global_Fx_Fy_Subsystem/1(Fx1) -> omega_alpha_and_k_values_subsystem/12(Fx1), F_M_subsystem/1(Fx1)  "Fx1"
  local_to_global_Fx_Fy_Subsystem/2(Fx2) -> omega_alpha_and_k_values_subsystem/13(Fx2), F_M_subsystem/2(Fx2)  "Fx2"
  local_to_global_Fx_Fy_Subsystem/3(Fx3) -> F_M_subsystem/3(Fx3), omega_alpha_and_k_values_subsystem/14(Fx3)  "Fx3"
  local_to_global_Fx_Fy_Subsystem/4(Fx4) -> F_M_subsystem/4(Fx4), omega_alpha_and_k_values_subsystem/15(Fx4)  "Fx4"

== system ISController/Vehicle_Sim/Vehicle_model/F_M_subsystem ==
  Fx1 : Inport  OutDataTypeStr=double  SampleTime=Ts
  Fx2 : Inport  Port=2  OutDataTypeStr=double  SampleTime=Ts
  Fx3 : Inport  Port=3  OutDataTypeStr=double  SampleTime=Ts
  Fx4 : Inport  Port=4  OutDataTypeStr=double  SampleTime=Ts
  Fy1 : Inport  Port=5  OutDataTypeStr=double  SampleTime=Ts
  Fy2 : Inport  Port=6  OutDataTypeStr=double  SampleTime=Ts
  Fy3 : Inport  Port=7  OutDataTypeStr=double  SampleTime=Ts
  Fy4 : Inport  Port=8  OutDataTypeStr=double  SampleTime=Ts
  l_f : Inport  Port=9  OutDataTypeStr=double  SampleTime=Ts
  l_r : Inport  Port=10  OutDataTypeStr=double  SampleTime=Ts
  w : Inport  Port=11  OutDataTypeStr=double  SampleTime=Ts
  Add : Sum  Inputs=++++
  Add1 : Sum  Inputs=++++
  Add2 : Sum  Inputs=++--
  Add3 : Sum
  Add4 : Sum
  Product{,1..3} (4 alike) : Product
  Subtract : Sum  Inputs=+-
  Subtract1 : Sum
  FX : Outport
  FY : Outport  Port=2
  Mz : Outport  Port=3
  wires:
  Fy2/1 -> Add3/2, Add1/2  "Fy2"
  Fx3/1 -> Subtract1/1, Add/1
  Fx4/1 -> Subtract1/2, Add/2
  Fx1/1 -> Subtract/2, Add/3  "Fx1"
  Fx2/1 -> Subtract/1, Add/4  "Fx2"
  Add/1 -> FX/1
  Fy1/1 -> Add3/1, Add1/1  "Fy1"
  Fy3/1 -> Add4/1, Add1/3
  Fy4/1 -> Add4/2, Add1/4
  Add1/1 -> FY/1
  Add2/1 -> Mz/1
  Add3/1 -> Product/1
  l_f/1 -> Product/2
  Product/1 -> Add2/1
  Subtract/1 -> Product1/2
  w/1 -> Product3/2, Product1/1
  Product1/1 -> Add2/2
  Add4/1 -> Product2/1
  l_r/1 -> Product2/2
  Product2/1 -> Add2/3
  Subtract1/1 -> Product3/1
  Product3/1 -> Add2/4
